simulink model "dual_source_ev_charging"  (R2025b)
settings: Solver=FixedStepDiscrete  StartTime=0.0  StopTime=28800  FixedStep=60  RelTol=1e-3
settings Model: Creator=User1  LastModifiedBy=User1
settings DataIOCC: ReturnWorkspaceOutputs=off

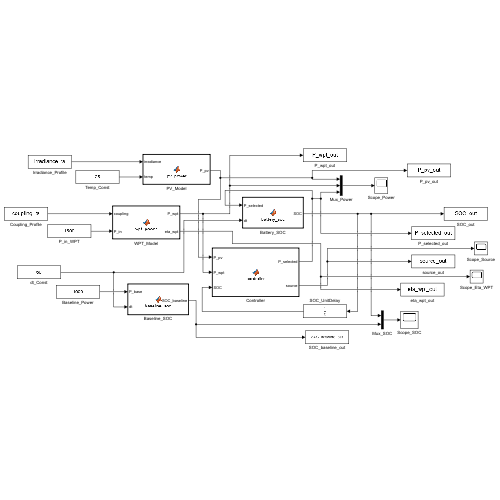
[thumbnail: Simulink's stored preview of the top-level diagram]
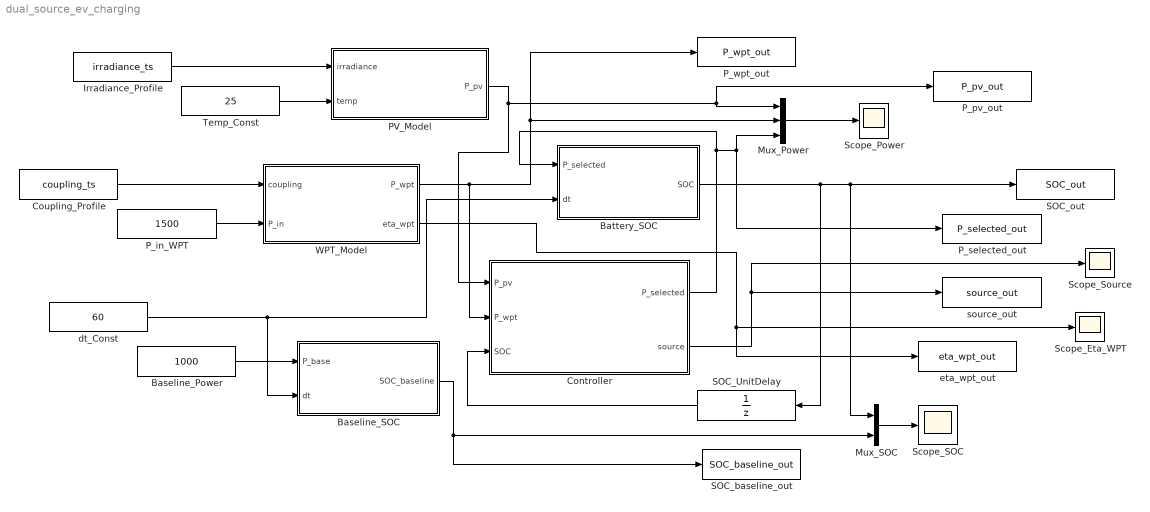
== system dual_source_ev_charging ==
  Baseline_Power : Constant  Value=1000
  Baseline_SOC : MATLAB Function  TreatAsAtomicUnit=on
  Battery_SOC : MATLAB Function  TreatAsAtomicUnit=on
  Controller : MATLAB Function  TreatAsAtomicUnit=on
  Coupling_Profile : FromWorkspace  VariableName=coupling_ts
  Irradiance_Profile : FromWorkspace  VariableName=irradiance_ts
  Mux_Power : Mux  Inputs=3
  Mux_SOC : Mux  Inputs=2
  PV_Model : MATLAB Function  TreatAsAtomicUnit=on
  P_in_WPT : Constant  Value=1500
  P_pv_out : ToWorkspace  VariableName=P_pv_out  SaveFormat=Structure With Time  SampleTime=-1
  P_selected_out : ToWorkspace  VariableName=P_selected_out  SaveFormat=Structure With Time  SampleTime=-1
  P_wpt_out : ToWorkspace  VariableName=P_wpt_out  SaveFormat=Structure With Time  SampleTime=-1
  SOC_UnitDelay : UnitDelay  SampleTime=60  HasFrameUpgradeWarning=on
  SOC_baseline_out : ToWorkspace  VariableName=SOC_baseline_out  SaveFormat=Structure With Time  SampleTime=-1
  SOC_out : ToWorkspace  VariableName=SOC_out  SaveFormat=Structure With Time  SampleTime=-1
  Scope_Eta_WPT : Scope
      settings: ActiveDisplayYMinimum=-1  ActiveDisplayYMaximum=1
  Scope_Power : Scope
      settings: ActiveDisplayYMinimum=-172.49999999999997  ActiveDisplayYMaximum=1552.5
  Scope_SOC : Scope
      settings: ActiveDisplayYMinimum=-1  ActiveDisplayYMaximum=1
  Scope_Source : Scope
      settings: ActiveDisplayYMinimum=0.875  ActiveDisplayYMaximum=2.125
  Temp_Const : Constant  Value=25
  WPT_Model : MATLAB Function  TreatAsAtomicUnit=on
  dt_Const : Constant  Value=60
  eta_wpt_out : ToWorkspace  VariableName=eta_wpt_out  SaveFormat=Structure With Time  SampleTime=-1
  source_out : ToWorkspace  VariableName=source_out  SaveFormat=Structure With Time  SampleTime=-1
  wires:
  Irradiance_Profile/1 -> PV_Model/1(irradiance)
  Temp_Const/1 -> PV_Model/2(temp)
  Coupling_Profile/1 -> WPT_Model/1(coupling)
  P_in_WPT/1 -> WPT_Model/2(P_in)
  PV_Model/1(P_pv) -> P_pv_out/1, Mux_Power/1, Controller/1(P_pv)
  WPT_Model/1(P_wpt) -> P_wpt_out/1, Mux_Power/2, Controller/2(P_wpt)
  SOC_UnitDelay/1 -> Controller/3(SOC)
  Controller/1(P_selected) -> P_selected_out/1, Mux_Power/3, Battery_SOC/1(P_selected)
  dt_Const/1 -> Battery_SOC/2(dt), Baseline_SOC/2(dt)
  Battery_SOC/1(SOC) -> SOC_out/1, Mux_SOC/1, SOC_UnitDelay/1
  Baseline_Power/1 -> Baseline_SOC/1(P_base)
  WPT_Model/2(eta_wpt) -> eta_wpt_out/1, Scope_Eta_WPT/1
  Controller/2(source) -> Scope_Source/1, source_out/1
  Baseline_SOC/1(SOC_baseline) -> SOC_baseline_out/1, Mux_SOC/2
  Mux_Power/1 -> Scope_Power/1
  Mux_SOC/1 -> Scope_SOC/1

== matlab function dual_source_ev_charging/WPT_Model ==
  data: coupling input; P_wpt output; P_in input; eta_wpt output
function [P_wpt, eta_wpt] = wpt_power(coupling, P_in)
    k0 = 0.3;
    eta_max = 0.92;
    eta_wpt = eta_max * (coupling/k0);
    eta_wpt = min(max(eta_wpt, 0), eta_max);
    P_wpt = P_in * eta_wpt;
end

== matlab function dual_source_ev_charging/PV_Model ==
  data: irradiance input; P_pv output; temp input
function P_pv = pv_power(irradiance, temp)
    G_ref = 1000;
    T_ref = 25;
    P_rated = 300;
    k_temp = -0.004;
    P_pv = P_rated * (irradiance/G_ref) * (1 + k_temp*(temp - T_ref));
    P_pv = max(P_pv, 0);
end

== matlab function dual_source_ev_charging/Controller ==
  data: P_pv input; P_selected output; P_wpt input; SOC input; source output
function [P_selected, source] = controller(P_pv, P_wpt, SOC)
    threshold = 100;
    if SOC >= 95
        P_selected = 0;
        source = 0;
    elseif P_pv > threshold
        P_selected = P_pv;
        source = 1;
    else
        P_selected = P_wpt;
        source = 2;
    end
end

== matlab function dual_source_ev_charging/Battery_SOC ==
  data: P_selected input; SOC output; dt input
function SOC = battery_soc(P_selected, dt)
    persistent E_stored
    if isempty(E_stored)
        E_stored = 0;
    end
    capacity_Wh = 40000;
    E_stored = E_stored + (P_selected * dt)/3600;
    E_stored = min(E_stored, capacity_Wh);
    SOC = (E_stored/capacity_Wh)*100;
end

== matlab function dual_source_ev_charging/Baseline_SOC ==
  data: P_base input; SOC_baseline output; dt input
function SOC_baseline = baseline_soc(P_base, dt)
    persistent E_stored
    if isempty(E_stored)
        E_stored = 0;
    end
    capacity_Wh = 40000;
    E_stored = E_stored + (P_base * dt)/3600;
    E_stored = min(E_stored, capacity_Wh);
    SOC_baseline = (E_stored/capacity_Wh)*100;
end
